simulink model "z8sim"  (R2016b)
settings: Solver=VariableStepAuto  StartTime=0.0  StopTime=20  RelTol=1e-3
values from neighbouring files (symbols this model uses):
  K = acker(A, B, p)    [z6.m]    (also in z7.m; z8.m)
  L = acker(A', C', [-1 -1 -1])    [z8.m]
  Nu = N(4)    [z7.m]    (also in z8.m)
  Nx = N(1:3)    [z7.m]    (also in z8.m)
  x0 = [0.1 0.1 0.1]    [z3.m]    (also in z6.m = [-1 2 1]; z7.m = [0 0 0]; z8.m = [-1 2 1])
undefined symbols (not defined in the file or in its folder): A, C
settings Model: Creator=E7440  LastModifiedBy=E7440

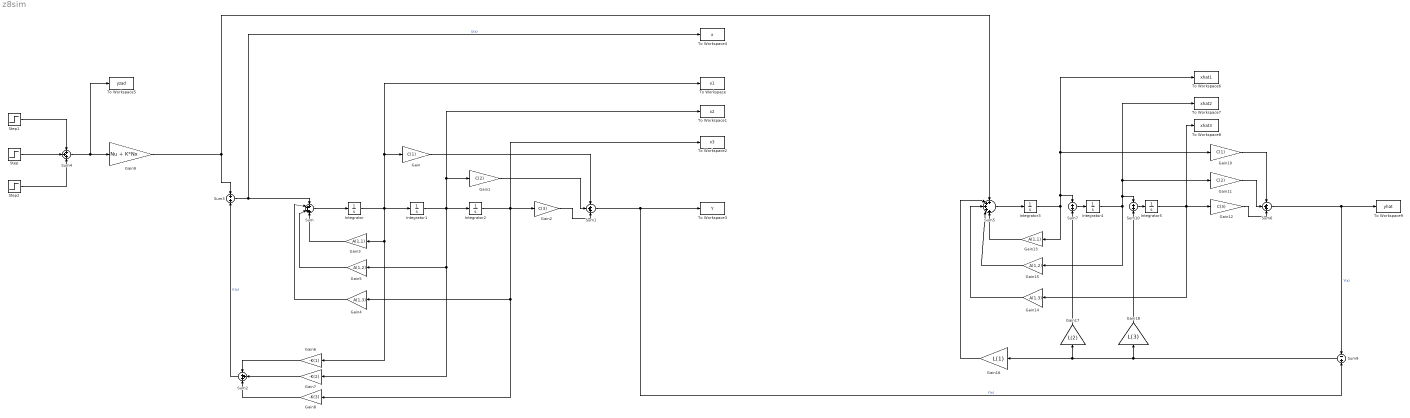
== system z8sim ==
  Gain : Gain  Gain=C(1)
  Gain1 : Gain  Gain=C(2)
  Gain10 : Gain  Gain=C(1)
  Gain11 : Gain  Gain=C(2)
  Gain12 : Gain  Gain=C(3)
  Gain13 : Gain  Gain=A(1,1)
  Gain14 : Gain  Gain=A(1,3)
  Gain15 : Gain  Gain=A(1,2)
  Gain16 : Gain  Gain=L(1)
  Gain17 : Gain  Gain=L(2)
  Gain18 : Gain  Gain=L(3)
  Gain2 : Gain  Gain=C(3)
  Gain3 : Gain  Gain=A(1,1)
  Gain4 : Gain  Gain=A(1,3)
  Gain5 : Gain  Gain=A(1,2)
  Gain6 : Gain  Gain=-K(1)
  Gain7 : Gain  Gain=-K(2)
  Gain8 : Gain  Gain=-K(3)
  Gain9 : Gain  Gain=Nu + K*Nx
  Integrator : Integrator  InitialCondition=x0(1)
  Integrator1 : Integrator  InitialCondition=x0(2)
  Integrator2 : Integrator  InitialCondition=x0(3)
  Integrator3 : Integrator  InitialCondition=x0(1)
  Integrator4 : Integrator  InitialCondition=x0(2)
  Integrator5 : Integrator  InitialCondition=x0(3)
  Step : Step  Time=10  SampleTime=0
  Step1 : Step  Time=4  After=-.5  SampleTime=0
  Step2 : Step  Time=15  After=-0.4  SampleTime=0
  Sum : Sum  Inputs=++++
  Sum1 : Sum  Inputs=+++
  Sum10 : Sum
  Sum2 : Sum  Inputs=3
  Sum3 : Sum
  Sum4 : Sum  Inputs=+++
  Sum5 : Sum  Inputs=+++++
  Sum6 : Sum  Inputs=+++
  Sum7 : Sum
  Sum9 : Sum  Inputs=-+
  To Workspace : ToWorkspace  VariableName=x1  SaveFormat=Timeseries  SampleTime=-1
  To Workspace1 : ToWorkspace  VariableName=x2  SaveFormat=Timeseries  SampleTime=-1
  To Workspace2 : ToWorkspace  VariableName=x3  SaveFormat=Timeseries  SampleTime=-1
  To Workspace3 : ToWorkspace  VariableName=Y  SaveFormat=Timeseries  SampleTime=-1
  To Workspace4 : ToWorkspace  VariableName=x  SaveFormat=Timeseries  SampleTime=-1
  To Workspace5 : ToWorkspace  VariableName=yzad  SaveFormat=Timeseries  SampleTime=-1
  To Workspace6 : ToWorkspace  VariableName=xhat1  SaveFormat=Timeseries  SampleTime=-1
  To Workspace7 : ToWorkspace  VariableName=xhat2  SaveFormat=Timeseries  SampleTime=-1
  To Workspace8 : ToWorkspace  VariableName=xhat3  SaveFormat=Timeseries  SampleTime=-1
  To Workspace9 : ToWorkspace  VariableName=yhat  SaveFormat=Timeseries  SampleTime=-1
  wires:
  Sum/1 -> Integrator/1
  Gain2/1 -> Sum1/3
  Gain1/1 -> Sum1/2
  Gain/1 -> Sum1/1
  Integrator2/1 -> To Workspace2/1, Gain8/1, Gain4/1, Gain2/1
  Integrator/1 -> Integrator1/1, Gain6/1, Gain3/1, To Workspace/1, Gain/1
  Gain3/1 -> Sum/4
  Integrator1/1 -> Integrator2/1, Gain7/1, Gain5/1, To Workspace1/1, Gain1/1
  Gain4/1 -> Sum/2
  Gain5/1 -> Sum/3
  Gain7/1 -> Sum2/2
  Gain6/1 -> Sum2/1
  Gain8/1 -> Sum2/3
  Sum2/1 -> Sum3/2  "K(s)"
  Sum3/1 -> To Workspace4/1, Sum/1  "U(s)"
  Sum5/1 -> Integrator3/1
  Gain12/1 -> Sum6/3
  Gain11/1 -> Sum6/2
  Gain10/1 -> Sum6/1
  Integrator5/1 -> To Workspace8/1, Gain14/1, Gain12/1
  Integrator3/1 -> To Workspace6/1, Gain10/1, Sum7/1, Gain13/1
  Gain13/1 -> Sum5/5
  Integrator4/1 -> Gain15/1, Sum10/1, To Workspace7/1, Gain11/1
  Gain14/1 -> Sum5/3
  Gain15/1 -> Sum5/4
  Sum6/1 -> To Workspace9/1, Sum9/1  "Y(s)"
  Sum1/1 -> Sum9/2, To Workspace3/1  "Y(s)"
  Sum9/1 -> Gain17/1, Gain16/1, Gain18/1
  Sum7/1 -> Integrator4/1
  Sum10/1 -> Integrator5/1
  Gain16/1 -> Sum5/2
  Gain17/1 -> Sum7/2
  Gain18/1 -> Sum10/2
  Gain9/1 -> Sum3/1, Sum5/1
  Step/1 -> Sum4/2
  Step1/1 -> Sum4/1
  Step2/1 -> Sum4/3
  Sum4/1 -> To Workspace5/1, Gain9/1
